simulink model "Acceleration"  (Simulink 8.7)
settings: Solver=VariableStepAuto  SolverMode=SingleTasking  StartTime=0.0  StopTime=30  FixedStep=0.1  RelTol=1e-3
values from neighbouring files (symbols this model uses):
  a = 31.111    [variabeln.m]
  b = -12.44444    [variabeln.m]
  Fz0 = 450*g    (= 4414.5)    [variabeln.m]
  g = 9.81    [variabeln.m]
  gear_ratio = 7.13    [variabeln.m]
  h_CoM = 0.5    [variabeln.m]
  J = 1    [variabeln.m]
  K_i = 1000    [variabeln.m]
  l = l_f+l_r    (= 3)    [variabeln.m]
  l_f = 1.5    [variabeln.m]
  lambda_target = 0.1    [variabeln.m]
  m = 700    [variabeln.m]
  max_torque = 140    [variabeln.m]
  Q = 1000    [variabeln.m]
  R = 0.01    [variabeln.m]
  r = 0.25    [variabeln.m]
  Ta0 = 800    [variabeln.m]
  theta1 = 0.86    [variabeln.m]
  theta2 = 33.82    [variabeln.m]
  theta3 = 0.35    [variabeln.m]
  W_luft = 0.5*cw*A*rho    (= 0.45)    [variabeln.m]
settings Model: Creator=frede  LastModifiedBy=Dominic
settings DataIOCC: ExternalInput=[t, u,m,g,r,J,theta1,theta2,theta3,v0,gear_ratio,v_max]  LimitDataPoints=off  SaveFormat=Dataset
settings DebuggingCC: UnderspecifiedInitializationDetection=Simplified  MergeDetectMultiDrivingBlocksExec=error  MaxConsecutiveZCsMsg=none  SFUnexpectedBacktrackingDiag=error  SFNoUnconditionalDefaultTransitionDiag=error
settings HardwareCC: ProdBitPerPointer=64  ProdLargestAtomicFloat=Float  ProdIntDivRoundTo=Zero  ProdEndianess=LittleEndian  ProdWordSize=64  ProdHWDeviceType=Intel->x86-64 (Windows64)
settings ModelReferenceCC: PropagateSignalLabelsOutOfModel=on
settings GRTTargetCC: TargetLangStandard=C99 (ISO)  GeneratePreprocessorConditionals=Use local settings
settings ConfigComp: CovMetricSettings=dwe  CovHtmlReporting=off  CovSaveCumulativeToWorkspaceVar=off  CovSaveSingleToWorkspaceVar=off  CovModelRefEnable=off  CovExternalEMLEnable=on

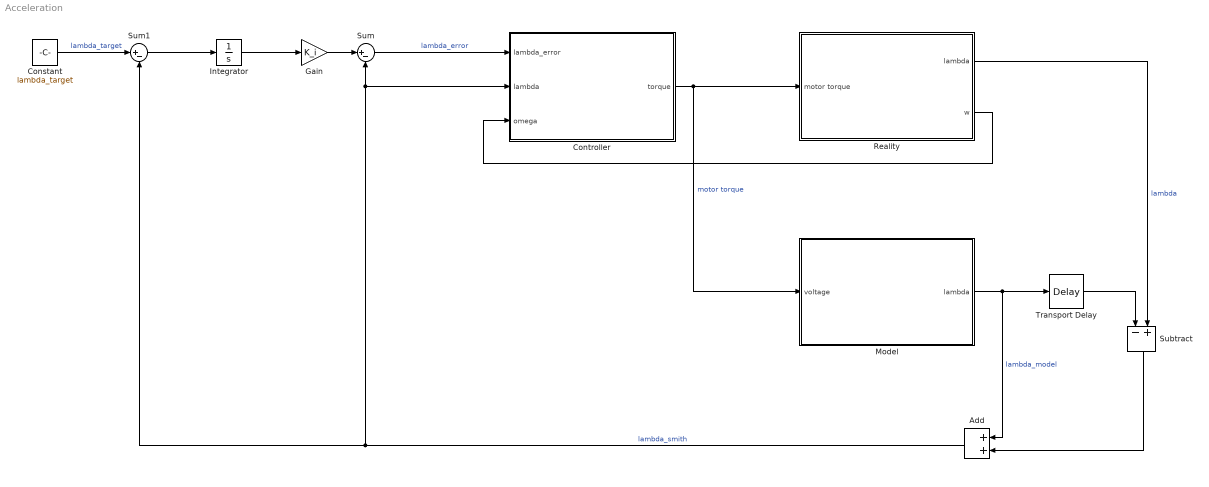
== system Acceleration ==
  Add : Sum  Inputs=2
  Constant : Constant  Value=lambda_target
  Controller : Subsystem
  Gain : Gain  Gain=K_i
  Integrator : Integrator
  Model : Subsystem
  Reality : Subsystem
  Subtract : Sum  Inputs=-+
  Sum : Sum  Inputs=|+-
  Sum1 : Sum  Inputs=|+-
  Transport Delay : TransportDelay  DelayTime=0.2
  wires:
  Sum/1 -> Controller/1(lambda_error)  "lambda_error"
  Controller/1(torque) -> Model/1(voltage), Reality/1(motor torque)  "motor torque"
  Reality/2(w) -> Controller/3(omega)
  Constant/1 -> Sum1/1  "lambda_target"
  Sum1/1 -> Integrator/1
  Model/1(lambda) -> Add/1, Transport Delay/1  "lambda_model"
  Add/1 -> Sum1/2, Controller/2(lambda), Sum/2  "lambda_smith"
  Transport Delay/1 -> Subtract/1
  Subtract/1 -> Add/2
  Gain/1 -> Sum/1
  Integrator/1 -> Gain/1
  Reality/1(lambda) -> Subtract/2  "lambda"

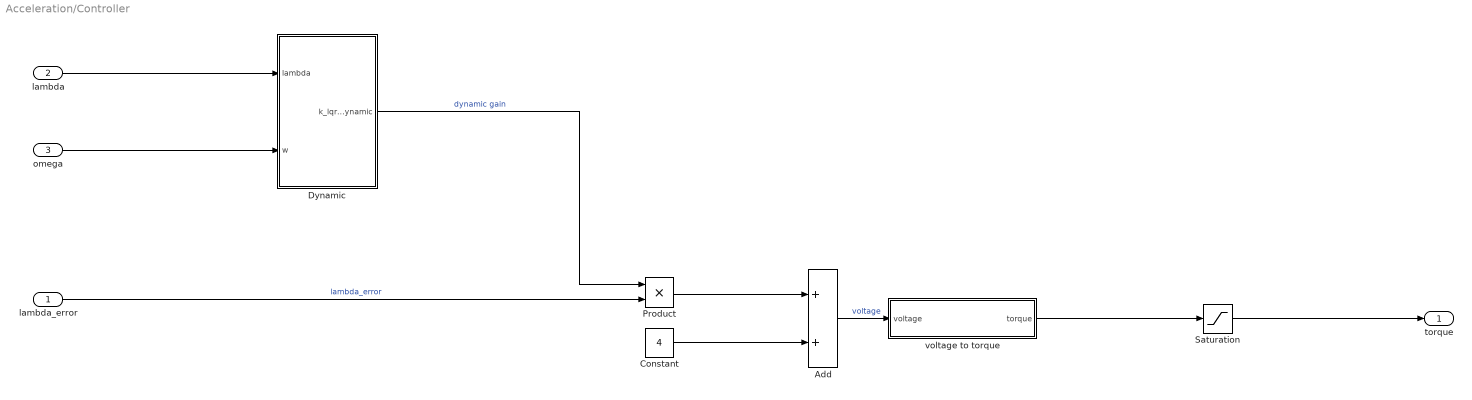
== system Acceleration/Controller ==
  lambda_error : Inport
  lambda : Inport  Port=2
  omega : Inport  Port=3
  Add : Sum
  Constant : Constant  Value=4
  Dynamic : MATLAB Function  TreatAsAtomicUnit=on
  Product : Product
  Saturation : Saturate  UpperLimit=max_torque  LowerLimit=0
  voltage to torque : MATLAB Function  TreatAsAtomicUnit=on
  torque : Outport
  wires:
  lambda/1 -> Dynamic/1(lambda)
  omega/1 -> Dynamic/2(w)
  Product/1 -> Add/1
  lambda_error/1 -> Product/2  "lambda_error"
  Constant/1 -> Add/2
  Dynamic/1(k_lqr_dynamic) -> Product/1  "dynamic gain"
  Add/1 -> voltage to torque/1(voltage)  "voltage"
  voltage to torque/1(torque) -> Saturation/1
  Saturation/1 -> torque/1

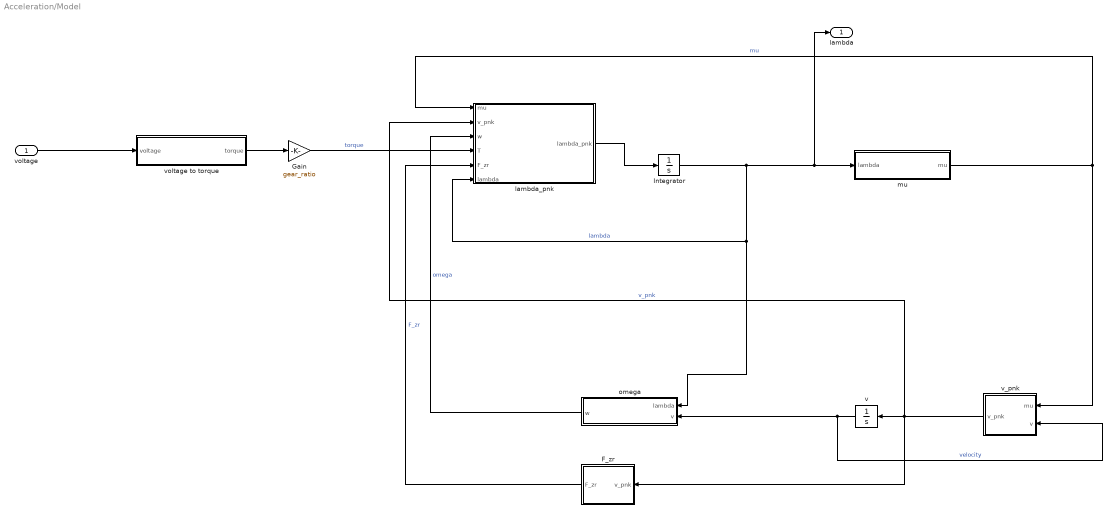
== system Acceleration/Model ==
  voltage : Inport
  F_zr : MATLAB Function  TreatAsAtomicUnit=on
  Gain : Gain  Gain=gear_ratio
  Integrator : Integrator
  lambda_pnk : MATLAB Function  TreatAsAtomicUnit=on
  mu : MATLAB Function  TreatAsAtomicUnit=on
  omega : MATLAB Function  TreatAsAtomicUnit=on
  v : Integrator  InitialCondition=0.1
  v_pnk : MATLAB Function  TreatAsAtomicUnit=on
  voltage to torque : MATLAB Function  TreatAsAtomicUnit=on
  lambda : Outport
  wires:
  Integrator/1 -> omega/1(lambda), lambda_pnk/6(lambda), lambda/1, mu/1(lambda)  "lambda"
  mu/1(mu) -> lambda_pnk/1(mu), v_pnk/1(mu)  "mu"
  v_pnk/1(v_pnk) -> lambda_pnk/2(v_pnk), v/1, F_zr/1(v_pnk)  "v_pnk"
  F_zr/1(F_zr) -> lambda_pnk/5(F_zr)  "F_zr"
  lambda_pnk/1(lambda_pnk) -> Integrator/1
  omega/1(w) -> lambda_pnk/3(w)  "omega"
  v/1 -> omega/2(v), v_pnk/2(v)  "velocity"
  voltage/1 -> voltage to torque/1(voltage)
  voltage to torque/1(torque) -> Gain/1
  Gain/1 -> lambda_pnk/4(T)  "torque"

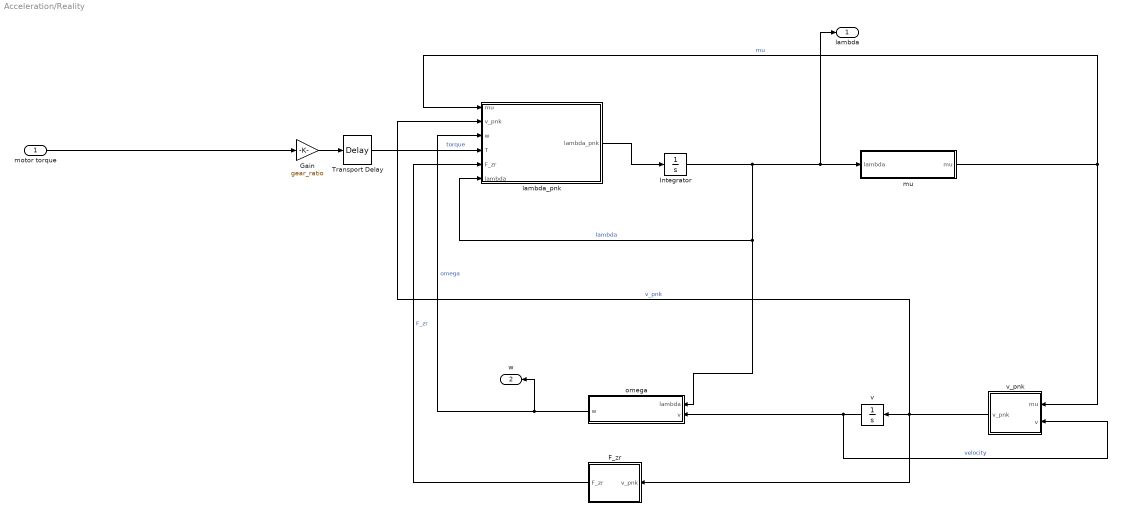
== system Acceleration/Reality ==
  motor torque : Inport
  F_zr : MATLAB Function  TreatAsAtomicUnit=on
  Gain : Gain  Gain=gear_ratio
  Integrator : Integrator
  Transport Delay : TransportDelay  DelayTime=0.2
  lambda_pnk : MATLAB Function  TreatAsAtomicUnit=on
  mu : MATLAB Function  TreatAsAtomicUnit=on
  omega : MATLAB Function  TreatAsAtomicUnit=on
  v : Integrator  InitialCondition=0.1
  v_pnk : MATLAB Function  TreatAsAtomicUnit=on
  lambda : Outport
  w : Outport  Port=2
  wires:
  Integrator/1 -> omega/1(lambda), lambda_pnk/6(lambda), lambda/1, mu/1(lambda)  "lambda"
  mu/1(mu) -> lambda_pnk/1(mu), v_pnk/1(mu)  "mu"
  v_pnk/1(v_pnk) -> lambda_pnk/2(v_pnk), v/1, F_zr/1(v_pnk)  "v_pnk"
  F_zr/1(F_zr) -> lambda_pnk/5(F_zr)  "F_zr"
  lambda_pnk/1(lambda_pnk) -> Integrator/1
  omega/1(w) -> w/1, lambda_pnk/3(w)  "omega"
  v/1 -> omega/2(v), v_pnk/2(v)  "velocity"
  motor torque/1 -> Gain/1
  Gain/1 -> Transport Delay/1
  Transport Delay/1 -> lambda_pnk/4(T)  "torque"

== matlab function Reality/mu ==
  data: lambda input double; mu output double; theta1 parameter double; theta2 parameter double; theta3 parameter double
function mu = mu(lambda, theta1, theta2, theta3)

if lambda>=0
    mu = theta1*(1-exp(-theta2*lambda))-lambda*theta3;
    
else
         mu = -(theta1*(1-exp(-theta2*abs(lambda)))-abs(lambda)*theta3);


end

== matlab function Model/F_zr ==
  data: F_zr output double; v_pnk input double; m parameter double; h_CoM parameter double; l parameter double; g parameter double; l_f parameter double
function F_zr = fcn(v_pnk,m, h_CoM, l, g, l_f)

F_zr=m*h_CoM/l*v_pnk+m*g*l_f/l;

end

== matlab function Reality/F_zr ==
  data: F_zr output double; v_pnk input double; m parameter double; h_CoM parameter double; l parameter double; g parameter double; l_f parameter double
function F_zr = fcn(v_pnk,m, h_CoM, l, g, l_f)

F_zr=m*h_CoM/l*v_pnk+m*g*l_f/l;

end

== matlab function Reality/lambda_pnk ==
  data: mu input double; v_pnk input double; lambda_pnk output double; w input double; T input double; F_zr input double; r parameter double; J parameter double; lambda input double
function lambda_pnk = fcn(mu,v_pnk,w,T,F_zr, r, J,lambda)

lambda_pnk=-v_pnk/(w*r)+(1-lambda)/w*T/J-(1-lambda)/w*r*F_zr*mu/J;

end

== matlab function Reality/omega ==
  data: lambda input double; v input double; w output double; r parameter double
function w = fcn(lambda, v,r)

w=v/(1-lambda)/r;

end

== matlab function Reality/v_pnk ==
  data: mu input double; v_pnk output double; g parameter double; l_f parameter double; l parameter double; h_CoM parameter double; v input double; W_luft parameter double; m parameter double
function v_pnk = fcn(mu,g, l_f, l, h_CoM,v,W_luft, m)

v_pnk=mu*g*l_f/(l-mu*h_CoM)-W_luft/((1-h_CoM/l*mu)*m)*v^2;

end

== matlab function Controller/Dynamic ==
  data: k_lqr_dynamic output double; lambda input double; w input double; m parameter double; r parameter double; J parameter double; theta1 parameter double; theta2 parameter double; theta3 parameter double; R parameter double; Q parameter double; Fz0 parameter double; Ta0 parameter double
function k_lqr_dynamic = fcn(lambda,w,m, r, J, theta1, theta2, theta3, R, Q, Fz0, Ta0)



A1=Ta0/(J*w)-Fz0*r/(J*w)*(theta1*theta2*exp(-lambda*theta2)-theta3)+Fz0*r/(J*w)*(theta1*(1-exp(-lambda*theta2)-lambda*theta2*exp(-lambda*theta2))-2*lambda*theta3)-Fz0/(m*r*w)*(theta1*theta2*exp(-lambda*theta2)-theta3);

B1=1/(J*w)-lambda/(J*w);


    k_lqr_dynamic =(A1+B1*sqrt(A1^2+B1^2*Q/R))/B1;

    
end

== matlab function Model/lambda_pnk ==
  data: mu input double; v_pnk input double; lambda_pnk output double; w input double; T input double; F_zr input double; r parameter double; J parameter double; lambda input double
function lambda_pnk = fcn(mu,v_pnk,w,T,F_zr, r, J,lambda)

lambda_pnk=-v_pnk/(w*r)+(1-lambda)/w*T/J-(1-lambda)/w*r*F_zr*mu/J;

end

== matlab function Model/mu ==
  data: lambda input double; mu output double; theta1 parameter double; theta2 parameter double; theta3 parameter double
function mu = mu(lambda, theta1, theta2, theta3)

if lambda>=0
    mu = theta1*(1-exp(-theta2*lambda))-lambda*theta3;
    
else
         mu = -(theta1*(1-exp(-theta2*abs(lambda)))-abs(lambda)*theta3);


end

== matlab function Model/omega ==
  data: lambda input double; v input double; w output double; r parameter double
function w = fcn(lambda, v,r)

w=v/(1-lambda)/r;

end

== matlab function Model/v_pnk ==
  data: mu input double; v_pnk output double; g parameter double; l_f parameter double; l parameter double; h_CoM parameter double; v input double; W_luft parameter double; m parameter double
function v_pnk = fcn(mu,g, l_f, l, h_CoM,v,W_luft, m)

v_pnk=mu*g*l_f/(l-mu*h_CoM)-W_luft/((1-h_CoM/l*mu)*m)*v^2;

end

== matlab function Model/voltage to torque ==
  data: voltage input double; torque output double; a parameter double; b parameter double
function torque = fcn(voltage,a, b)

torque = a*voltage+b;

== matlab function Controller/voltage to torque ==
  data: voltage input double; torque output double; a parameter double; b parameter double
function torque = fcn(voltage,a, b)

torque = a*voltage+b;
